simulink library "DriveStraight"  (R2018b)
settings: Solver=VariableStepAuto  StartTime=0.0  StopTime=10.0  RelTol=1e-3
settings Model: Creator=nico  LastModifiedBy=nico

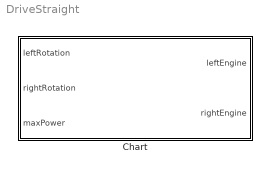
== system DriveStraight ==
  Chart : Stateflow chart  TreatAsAtomicUnit=on

== stateflow chart DriveStraight/Chart ==
  state StartDriving
    entry: leftEngine = maxPower
    entry: rightEngine = maxPower
    entry: leftOffset = leftRotation
    entry: rightOffset = rightRotation
  state StartCorrection
    diff=(leftRotation-leftOffset) - (rightRotation-rightOffset)
  state TurnRight
  state TurnLeft
  state IncreaseLeft
    entry: leftEngine = leftEngine + correctionStep
  state IncreaseRight
    entry: rightEngine = rightEngine + correctionStep
  state DecreaseLeft
    entry: leftEngine = leftEngine - correctionStep
  state DecreaseRight
    entry: rightEngine = rightEngine - correctionStep
  (default) -> StartDriving
  StartDriving -> StartCorrection
  StartCorrection -> TurnRight [order 2] : [diff < -threshold]
  StartCorrection -> TurnLeft [order 1] : [diff > threshold]
  TurnRight -> StartCorrection [order 3] : [rightEngine<maxPower]
  TurnRight -> IncreaseLeft [order 2] : [leftEngine < maxPower]
  TurnRight -> DecreaseRight [order 1] : [leftEngine==maxPower && rightEngine==maxPower]
  TurnLeft -> StartCorrection [order 3] : [leftEngine<maxPower]
  TurnLeft -> DecreaseLeft [order 2] : [rightEngine==maxPower && leftEngine==maxPower]
  TurnLeft -> IncreaseRight [order 1] : [rightEngine<maxPower]
  IncreaseRight -> StartCorrection
  DecreaseLeft -> StartCorrection
  DecreaseRight -> StartCorrection
  IncreaseLeft -> StartCorrection
  data: leftEngine output int32; rightEngine output int32; leftRotation input; rightRotation input; leftOffset local; rightOffset local; diff local int32; correctionStep constant int32 =1; threshold constant int32 =1; maxPower input int32 =100
